simulink model "lorenz"  (R2017b)
settings: Solver=ode4  StartTime=0.0  StopTime=120  FixedStep=0.002  RelTol=1e-3
settings Model: Creator=squirrel  LastModifiedBy=squirrel

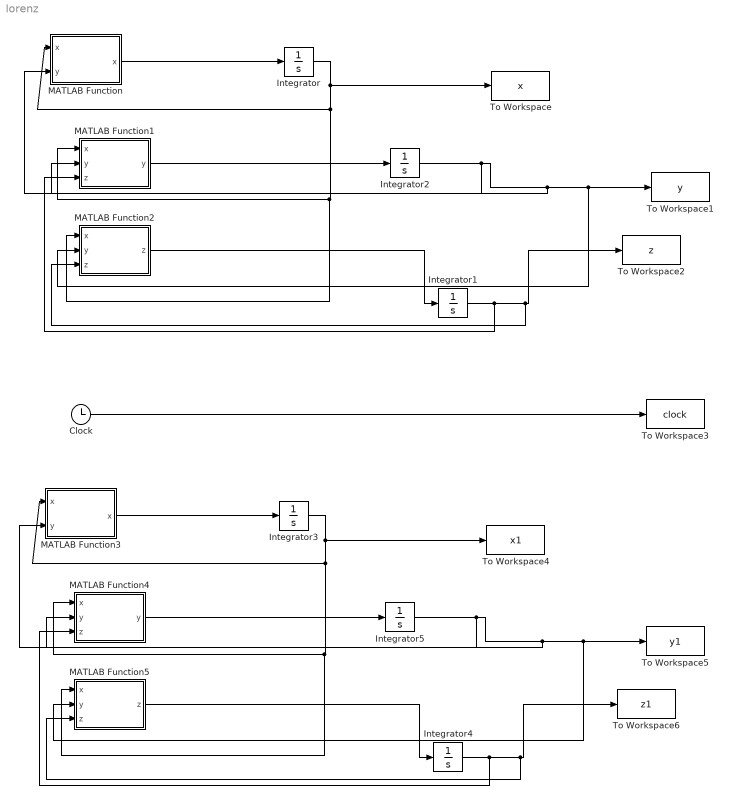
== system lorenz ==
  Clock : Clock
  Integrator{,2..3,5} (4 alike) : Integrator  InitialCondition=0.01
  Integrator1 : Integrator
  Integrator4 : Integrator
  MATLAB Function : MATLAB Function  TreatAsAtomicUnit=on
  MATLAB Function1 : MATLAB Function  TreatAsAtomicUnit=on
  MATLAB Function2 : MATLAB Function  TreatAsAtomicUnit=on
  MATLAB Function3 : MATLAB Function  TreatAsAtomicUnit=on
  MATLAB Function4 : MATLAB Function  TreatAsAtomicUnit=on
  MATLAB Function5 : MATLAB Function  TreatAsAtomicUnit=on
  To Workspace : ToWorkspace  VariableName=x  SampleTime=-1
  To Workspace1 : ToWorkspace  VariableName=y  SampleTime=-1
  To Workspace2 : ToWorkspace  VariableName=z  SampleTime=-1
  To Workspace3 : ToWorkspace  VariableName=clock  SampleTime=-1
  To Workspace4 : ToWorkspace  VariableName=x1  SampleTime=-1
  To Workspace5 : ToWorkspace  VariableName=y1  SampleTime=-1
  To Workspace6 : ToWorkspace  VariableName=z1  SampleTime=-1
  wires:
  MATLAB Function/1(x) -> Integrator/1
  MATLAB Function1/1(y) -> Integrator2/1
  MATLAB Function2/1(z) -> Integrator1/1
  Clock/1 -> To Workspace3/1
  Integrator/1 -> MATLAB Function/1("x "), MATLAB Function2/1(x), MATLAB Function1/1(x), To Workspace/1
  Integrator2/1 -> MATLAB Function/2(y), MATLAB Function1/2("y "), MATLAB Function2/2(y), To Workspace1/1
  Integrator1/1 -> MATLAB Function1/3(z), MATLAB Function2/3("z "), To Workspace2/1
  Integrator5/1 -> MATLAB Function3/2(y), MATLAB Function4/2("y "), MATLAB Function5/2(y), To Workspace5/1
  MATLAB Function5/1(z) -> Integrator4/1
  MATLAB Function3/1(x) -> Integrator3/1
  Integrator4/1 -> MATLAB Function4/3(z), MATLAB Function5/3("z "), To Workspace6/1
  Integrator3/1 -> MATLAB Function3/1("x "), MATLAB Function5/1(x), MATLAB Function4/1(x), To Workspace4/1
  MATLAB Function4/1(y) -> Integrator5/1

== matlab function lorenz/MATLAB Function1 ==
  data: x input; y output; y input; z input
function y = Y(x, y, z)

y = (40 -z) * x - y;

== matlab function lorenz/MATLAB Function ==
  data: x input; x output; y input
function x = X(x, y)

x = -10 * (x - y);

== matlab function lorenz/MATLAB Function2 ==
  data: x input; z output; y input; z input
function z = Z(x, y, z)

z = x * y - 2.67 * z;

== matlab function lorenz/MATLAB Function3 ==
  data: x input; x output; y input
function x = X(x, y)

x = -10 * (x - y);

== matlab function lorenz/MATLAB Function4 ==
  data: x input; y output; y input; z input
function y = Y(x, y, z)

y = (40.000000001 -z) * x - y;

== matlab function lorenz/MATLAB Function5 ==
  data: x input; z output; y input; z input
function z = Z(x, y, z)

z = x * y - 2.67 * z;
